simulink model "Expriment_Gaze"  (R2014a)
settings: Solver=FixedStepDiscrete  SolverMode=SingleTasking  StartTime=0.0  StopTime=inf  FixedStep=0.01  RelTol=1e-3
PostLoadFcn:
  | h_RPStest = RPStest;
model workspace (MAT data in the model file):
  gtest = 0
undefined symbols (not defined in the file or in its folder): avert, avert_freq_factor, avert_gaze_dirs_chance, avert_gaze_duration_factor, avert_head_frequency_factor, avert_head_speed, BML, BML1, BML2, bmlsL, bmlsM, bodyBusyFlag, clock, emotion_amount_factor, faceBusyFlag, fileID, GAZE_WIN, gazing, mut_freq_factor, mutual_gaze_duration_factor, P, pose_cat_chance, pose_chanc_factor, pose_chance_factor, pose_frequency_factor, pose_lean, pose_lean_flag, pose_speed, pose_twitch, pr, serial, STATE_BEFORE, STATE_GO, STATE_OVER, STATE_READY, Stateflow
libraries: simulink x24, instrumentlib x6, lib_affectiveChar_behavior x3, realtime_pacer_lib x2, lib_affectiveChar_input x1
(part 7 of 7)

== stateflow chart Expriment_Gaze/CharacterControl/facialExpression_Controller ==
  state subSmile [parallel]
    settings: executionOrder=1
    state stateInitial
      entry: avert=1; gameState=14;
      n=encStr2Arr(' ');bmlsM=[n n n n n];newBmlsM=[n n n n n];
    state stateCheckSmile
    state gazeCamera
      entry:  [P,BMLM]= smileTable(2) ;avert=0;
      newBmlsM=insertQueue(bmlsM,BMLM);
      bmlsM=newBmlsM;
    state wait
    state checkP
      entry:  [P,BMLM]=  smileTable(1) ;
      newBmlsM=insertQueue(bmlsM,BMLM);
      bmlsM=newBmlsM;
    (default) -> stateInitial
    stateInitial -> stateCheckSmile : [gameState==20]
    stateCheckSmile -> stateCheckSmile [order 2]
    gazeCamera -> stateCheckSmile [order 2] : after(1,secs)[isSmiling~=1]
    wait -> stateCheckSmile : after(10,secs)
    stateCheckSmile -> gazeCamera [order 1] : [[isSmiling==1]&[ gameState~= STATE_GO]&[ gameState~= STATE_READY]]
    checkP -> wait
    gazeCamera -> checkP [order 1] : after(1,secs)[isSmiling==1]
  note: SMILE_DUER=10 seceonds
  note: check if still isSmiling is true works as a buffer to remove the smiles that last ony 1 sec (system errors).
  state subFacial [parallel]
    settings: executionOrder=2
    state stateFacialExpression
      entry:
      emotion_amount_factor =set_AU_Amount(inA,inV,personality);
      BMLl=cmdBML_AU_VA(emotion_amount_factor);
      newBmlsL=insertQueueLow(bmlsL,BMLl); bmlsL=newBmlsL;
    state initial
    state wait3
    (default) -> initial
    initial -> stateFacialExpression : [gameState==20]
    wait3 -> stateFacialExpression : after(7,secs)
    stateFacialExpression -> wait3
  data: bmls function_input double size=[1000,5]; myBML function_input double size=[1000,1]; newBmls function_output double size=[1000,5]; bmls function_input double size=[1000,5]; myBML function_input double size=[1000,1]; newBmls function_output double size=[1000,5]; bmlID function_input double; p function_output double size=1; poseBML function_output double size=[1000,1]; bmlID function_input double; p function_output double size=1; poseBML function_output double size=[1000,1]; eAmountFactor function_output double size=[1,11]; arousal function_input double size=1; valence function_input double size=1; inPersonality function_input double size=1; smileN local double size=1; isSmiling input double size=1 =0; avert data_store_memory =0; gazing data_store_memory size=2; GAZE_WIN data_store_memory size=2; BML data_store_memory size=[256,1]; P data_store_memory; fileID local double size=1; gameState output double; STATE_GO data_store_memory; STATE_READY data_store_memory; STATE_BEFORE data_store_memory; newBmlsM local double size=[1000,5]; bmlsM data_store_memory size=[256,1]; BMLM local double size=[1000,1]; n local; personality input double size=1; internalE input double size=1; au local; emotion_amount_factor data_store_memory; aChange input boolean size=1; au_i local double size=1; au_L local double size=1; emoDisp local; bmlsL data_store_memory size=[256,1]; BMLl local double size=[1000,1]; newBmlsL local double size=[1000,5]; emotion_amount_custom input double size=1; inA input double size=1; inV input double size=1; vChange input boolean size=1
  events: secs input RISING_EDGE_EVENT
  function newBmls =insertQueue(bmls,myBML):
    | function newBmls =insertQueue(bmls,myBML)
    |     full=1;
    |     t=encStr2Arr(' ');
    |     newBmls=[t t t t t];
    |     for i = 1:5
    |         if (isequal(bmls(:,i),t))
    |             %add to end of the queue where its empty
    |             bmls(:,i)=myBML;
    |             full=0;
    |             break
    |         end
    |     end
    |     if(full~=0)
    |             %if queue full, shift all elements to left which removes the first one, then add to end
    |             bmls(:,1)= bmls(:,2);
    |             bmls(:,2)= bmls(:,3);
    |             bmls(:,3)= bmls(:,4);
    |             bmls(:,5)=myBML;
    |     end
    |     newBmls=bmls;
  function newBmls =insertQueueLow(bmls,myBML):
    | function newBmls =insertQueueLow(bmls,myBML)
    |     full=1;
    |     t=encStr2Arr(' ');
    |     newBmls=[t t t t t];
    |     for i = 1:5
    |         if (isequal(bmls(:,i),t))
    |             %add to end of the queue where its empty
    |             bmls(:,i)=myBML;
    |             full=0;
    |             break
    |         end
    |     end
    |     if(full~=0)
    |             %if queue full, shift all elements to left which removes the first one, then add to end
    |             bmls(:,1)= bmls(:,2);
    |             bmls(:,2)= bmls(:,3);
    |             bmls(:,3)= bmls(:,4);
    |             bmls(:,5)=myBML;
    |     end
    |     newBmls=bmls;
  function [p,poseBML] = smileTable(bmlID):
    | function [p,poseBML] = smileTable(bmlID)
    | 
    | aVarTruthTableCondition_1 = false;
    | aVarTruthTableCondition_2 = false;
    | 
    | 
    | % smile
    | 
    | aVarTruthTableCondition_1 = logical(bmlID==1);
    | 
    | % headN
    | 
    | aVarTruthTableCondition_2 = logical(bmlID==2);
    | 
    | if (aVarTruthTableCondition_1)
    |     aFcnTruthTableAction_1();
    | elseif (aVarTruthTableCondition_2)
    |     aFcnTruthTableAction_2();
    | else % Default
    |     aFcnTruthTableAction_1();
    | end
    | 
    | function aFcnTruthTableAction_1()
    | 
    | % smile
    | 
    | poseBML=encStr2Arr('<?xml version="1.0"?><act><bml><face amount="1" au="12" side="BOTH" start="0" stroke="2" relax="3" end="4" type="facs"/><face amount="0.3" au="6" side="BOTH" start="0" stroke="2" relax="3" end="4" type="facs"/></bml></act>');p=3;
    | 
    | function aFcnTruthTableAction_2()
    | 
    | % headNeutralBrow
    | 
    | poseBML=encStr2Arr('<?xml version="1.0" ?><act><bml><gaze target="gazeTarget" start="0" end="5" sbm:time-hint="1.5"/></bml></act>');p=3;
    | 
    | function aFcnTruthTableAction_3()
    | 
    | % smileBrow
    | 
    | poseBML=encStr2Arr('<?xml version="1.0"?><act><bml><face amount="0.1" au="1" side="BOTH" start="0" stroke="2" relax="4" end="6" type="facs"/><face amount="0.1" au="2" side="BOTH" start="0" stroke="2" relax="4" end="6" type="facs"/></bml></act>');p=3;
  function [p,poseBML] = facialExpr(bmlID):
    | function [p,poseBML] = facialExpr(bmlID)
    | 
    | aVarTruthTableCondition_1 = false;
    | aVarTruthTableCondition_2 = false;
    | 
    | 
    | % smile
    | 
    | aVarTruthTableCondition_1 = logical(bmlID==1);
    | 
    | % headN
    | 
    | aVarTruthTableCondition_2 = logical(bmlID==2);
    | 
    | if (aVarTruthTableCondition_1)
    |     aFcnTruthTableAction_1();
    | elseif (aVarTruthTableCondition_2)
    |     aFcnTruthTableAction_2();
    | else % Default
    |     aFcnTruthTableAction_1();
    | end
    | 
    | function aFcnTruthTableAction_1()
    | 
    | % smile
    | 
    | poseBML=encStr2Arr('<?xml version="1.0"?><act><bml><face amount="1" au="12" side="BOTH" start="0" stroke="10" relax="70" end="100" type="facs"/><face amount="0.3" au="6" side="BOTH" start="0" stroke="10" relax="70" end="100" type="facs"/></bml></act>');p=3;
    | 
    | function aFcnTruthTableAction_2()
    | 
    | % headNeutralBrow
    | 
    | poseBML=encStr2Arr('<?xml version="1.0" ?><act><bml><gaze target="gazeTarget" start="0" end="5" sbm:time-hint="1.5"/></bml></act>');p=3;
    | 
    | function aFcnTruthTableAction_3()
    | 
    | % smileBrow
    | 
    | poseBML=encStr2Arr('<?xml version="1.0"?><act><bml><face amount="0.1" au="1" side="BOTH" start="0" stroke="2" relax="4" end="6" type="facs"/><face amount="0.1" au="2" side="BOTH" start="0" stroke="2" relax="4" end="6" type="facs"/></bml></act>');p=3;
  function eAmountFactor  =set_AU_Amount(arousal,valence,inPersonality):
    | function eAmountFactor  =set_AU_Amount(arousal,valence,inPersonality)
    | %     15-12-2015, PAD drivern facial expr simul, Grammer data to map AU and VA
    | %     fprintf('VA: %0.0f,%0.0f\r\n',arousal,valence);
    | %     scale
    | %     p = valence * (20/9)  - 10;
    | %     a = arousal * (20/9)  - 10;
    | 
    |     p=valence;a=arousal;
    |     all_AUs=[1,2,4,5,6, 7,12,26,45,10, 25];eAmountFactor=[0,0,0,0,0, 0,0,0,0,0, 0];
    |     for c=1:11
    |         eAmountFactor(1)=0.003*p-0.002*a;  %1,-0.002*a
    |         eAmountFactor(2)=-0.002*p+0.010*a; %2,+0.010*a
    | %         eAmountFactor(12)=-0.016*p+0.034*a; %27 moth open stretch
    |         eAmountFactor(8)=-0.002*p+0.023*a;  %26,-0.002*p+0.049*a
    |         eAmountFactor(5)=-0.008*p+0.009*a;  %6
    |         
    | %         eAmountFactor(13)=0.002*p+0.004*a; %18 lip Puckerer, W 0.3=101
    | %         eAmountFactor(14)=0.007*p+0.025*a; %22 lip fumeler, ShCh 0.5=102       
    | %         eAmountFactor(15)=0.003*p+0.009*a; %14 dimpler FV+PBM 0.5=103
    | %         eAmountFactor(16)=0.003*p+0.009*a; %14 dimpler FV+PBM 0.5=103
    | %         eAmountFactor=-0.010*p+0.017*a;  %17 chin raiser
    | 
    |         eAmountFactor(10)=-0.020*p+0.020*a;  %10 upper lip raiser,-0.053*p+0.026*a
    |         eAmountFactor(4)=-0.003*p+0.032*a; %5 upper lid raiser
    |         eAmountFactor(9)=-0.011*p-0.011*a; %eye closed, 45 instead of 43,-0.021*p-0.037*a
    |         eAmountFactor(3)=-0.036*p+0.022*a; %4 brow lowerer
    | %       eAmountFactor=-0.008*p+0.006*a;    %9 nose wrikler ,10
    | %       eAmountFactor=-0.004*p+0.004*a;    %39?
    | %       eAmountFactor=-0.010*p+0.008*a;    %38?
    | 
    |         eAmountFactor(11)=-0.011*p+0.023*a;%25 lip open,-0.023*p+0.058*a
    | %       eAmountFactor(17)=-0.004*p-0.003*a;    %24 lip pressor, PBM =104       
    | %       eAmountFactor(18)=-0.011*p+0.009*a;    %23 lip tightner PBM0.2 + W0.6=105
    | %       eAmountFactor(19)=-0.011*p+0.009*a;    %23 lip tightner PBM0.2 + W0.6=105
    | 
    | %       eAmountFactor=-0.004*p+0.003*a;    %19?
    | 
    | %       eAmountFactor(20)=0.039*p+0.015*a;  %13 cheek puffer, W 0.3 =106
    |         
    |         eAmountFactor(6)=-0.005*p-0.001*a; %7  Lid Tightener
    |         eAmountFactor(7)=0.057*p+0.009*a;  %12 Lip Corner Puller
    |     %   eAmountFactor=-0.008*p+0.009*a;    %11 Nasolabial Deepener
    |     %   eAmountFactor=-0.046*p-0.002*a;    %15 Lip Corner Depressor
    |     %   eAmountFactor=-0.014*p+0.016*a;    %16 Lower Lip Depressor
    |     %   eAmountFactor(20)=-0.026*p+0.010*a;%20 lip stretch
    |         
    |         eAmountFactor=eAmountFactor/6; %scale
    |         if(inPersonality==2 || inPersonality==4)%introvert
    |             eAmountFactor=eAmountFactor/1.3; % divide by 4/3
    |         end
    |     end

== stateflow chart Expriment_Gaze/GazeFollowSubsystem/reactiveGaze/createGazePawn ==
  state sendBML(In1) [function]
  state sendSBM(In2) [function]
  state stateCreatePawn
    entry:
    sendSBM( encStr2Arr( 'gt = scene.createPawn("gazeTarget")' ) );
    sendBML(encStr2Arr('<?xml version="1.0" ?><act><bml><gaze sbm:joint-range="EYES BACK" target="gazeTarget"/></bml></act>'));
  (default) -> stateCreatePawn
  data: In1 function_input double size=[1000 1]; In2 function_input double size=[1000 1]

== matlab function Expriment_Gaze/randomArray/makleArray ==
  data: r1 input; y output double size=[1,25]; r2 input; r3 input; r4 input; r5 input; r6 input; r7 input; r8 input; r9 input; r10 input; r11 input; r12 input; r13 input; r14 input; r15 input; r16 input; r17 input; r18 input; r19 input; r20 input; r21 input; r22 input; r23 input; r24 input; r25 input
function y = fcn(r1,r2,r3,r4,r5,r6,r7,r8,r9,r10,r11,r12,r13,r14,r15,r16, r17, r18, r19,r20,r21,r22,r23,r24,r25)
%#codegen
y=[0,0,0,0,0,0,0,0,0,0,0,0,0,0,0,0,0,0,0,0,0,0,0,0,0];
y(:,1) = floor(r1);
y(:,2) = floor(r2);
y(:,3) = floor(r3);
y(:,4) = floor(r4);
y(:,5) = floor(r5);
y(:,6) = floor(r6);
y(:,7) = floor(r7);
y(:,8) = floor(r8);
y(:,9) = floor(r9);
y(:,10) = floor(r10);
y(:,11) = floor(r11);
y(:,12) = floor(r12);
y(:,13) = floor(r13);
y(:,14) = floor(r14);
y(:,15) = floor(r15);
y(:,16) = floor(r16);
y(:,17) = floor(r17);
y(:,18) = floor(r18);
y(:,19) = floor(r19);
y(:,20) = floor(r20);
y(:,21) = floor(r21);
y(:,22) = floor(r22);
y(:,23) = floor(r23);
y(:,24) = floor(r24);
y(:,25) = floor(r25);

== matlab function Expriment_Gaze/GazeFollowSubsystem/gazeFollow ==
  data: state input; stateOver output
function stateOver = fcn(state)
%#codegen

%Maryam 30/06/2015
%Here set in which states of the interaction agent experienced 
% more arousal(arousalFlag=1) and less arousal (arousalFlag=-1)

%Note that you should define the states in your scenraio beforehand

%we assume agent gets more aroused when in ready/go state and 
%less aroused when in WAITE/HAND

if(state==3)%only gaze follows user in ganme-over states 
                      %since in other states we assume user is not moving
    stateOver=1;
else
    stateOver=0;

end

== matlab function Expriment_Gaze/handUpTable ==
  data: R input; L input; y output
function y = fcn(R, L)

aVarTruthTableCondition_1 = false;
aVarTruthTableCondition_2 = false;
aVarTruthTableCondition_3 = false;
aVarTruthTableCondition_4 = false;


% no hand up

aVarTruthTableCondition_1 = logical(R==0 && L==0);

% right hand up

aVarTruthTableCondition_2 = logical(R==1 && L==0);

% left hand up

aVarTruthTableCondition_3 = logical(R==0 && L==1);

% both hands up

aVarTruthTableCondition_4 = logical(R==1 && L==1);

if (aVarTruthTableCondition_1)
    aFcnTruthTableAction_1();
elseif (aVarTruthTableCondition_2)
    aFcnTruthTableAction_2();
elseif (aVarTruthTableCondition_3)
    aFcnTruthTableAction_3();
elseif (aVarTruthTableCondition_4)
    aFcnTruthTableAction_4();
else % Default
    aFcnTruthTableAction_1();
end

function aFcnTruthTableAction_1()

% no hand up

y = 0;

function aFcnTruthTableAction_2()

% right hand up

y = 1;

function aFcnTruthTableAction_3()

% left hand up

y = 2;

function aFcnTruthTableAction_4()

% both hands up

y = 3;

== matlab function Expriment_Gaze/facialExpr/facialExprGen/setAU ==
  data: E input double size=1; AU output double size=[1,6]; L output double size=1
function [AU,L]=setAU(E)	
% 1	Inner Brow Raiser,% 2	Outer Brow Raiser, % 4	Brow Lowerer
% 5	Upper Lid Raiser,% 6	Cheek Raiser,% 7	Lid Tightener
% 8	Lips Toward Each Other,% 9	Nose Wrinkler,% 10	Upper Lip Raiser	
% 11	Nasolabial Deepener	% 12	Lip Corner Puller % 13	Sharp Lip Puller % 14	Dimpler	
% 15	Lip Corner Depressor % 16	Lower Lip Depressor % 17	Chin Raiser	mentalis
% 18	Lip Pucker	% 19	Tongue Show	% 20	Lip Stretcher % 21	Neck Tightener	platysma
% 22	Lip Funneler% 23	Lip Tightener% 24	Lip Pressor % 25	Lips Part	depressor
% 26	Jaw Drop,% 27	Mouth Stretch
% 43	Eyes Closed, % 44	Eyebrow Gatherer,% 45	Blink,% 46	Wink
%smartbody no 43,15,17,10 looks wierd,no 142
   AU=[6,12,142,0,0,0];L=3;
   % AU5(eyeOpen) for A+
   % AU1,4 for V-
   %AU12 for V+
    switch(E)
        case 1 %V- A-,bored (43)[1]
            AU=[1,2,45,0,0,0];L=3;%[1,1,0.35]
        
        case 2 %V- A-;sad %(1,2,4,10,15,17,43)[];can be [1,2,4,45,6,0]
            AU=[1,4,0,0,0,0];L=2;%[1,1,0,0,0,0]
        
        case 3 %V- A+,frust(2,1,14)[1],(-1,-2,4,7,14)[2], maybe(1,7)[0.7,0.7,0.5]
            AU=[1,2,4,5,6,0];L=5;%[1,1,1,0.5,0.5,0]
        
        case 4 %V- A+,fear(1,2,4,5,25=mouth)
            AU=[1,2,4,5,6,7];L=6; %[1,1,1,0.2,0.2]
        
        case 5%V+ A-,calm,sleepy
            AU=[12,14,0,0,0,0];L=2;%[0.7,0.3,0,0,0,0]
        
        case 7%V+ A+,happy
            AU=[6,12,0,0,0,0];L=2;%[1,0.5,0,0,0,0]
        
        case 8%V+ A+,excited
            AU=[12,26,5,1,2,0];L=5;%[1,1,1,1,1,0]
        
        case 9%V- A+, angry
            AU=[2,4,5,7,45,0];L=5;%[0.5,1,0.2,0.2,0.2]
        
        otherwise
            %confusion (1,2,4,7)[1] %[1,1,1,0.2]
            %worried (1,2,4,5) [1,1,1,0.5]
            %angry(4,5,7,10,27)[], can be(2,4,5,7,45)[0.5,1,0.2,0.2,0.2]

            AU=[4,7,12,0,0,0];L=3;
            disp('error, emotion not listed:');disp(E);
    end  
%[1]Craig S.D. et al(2004)emotions during learning:the first steps tw affect sensitive
%[2]grafsgard J F () automatically recog facial indicator of frust

== matlab function Expriment_Gaze/facialExpr/facialExprGen/forloop/displayBMLs ==
  data: e input; l input; i input double size=1 [1..]; bml input
function fcn(e,l,i,bml)
%#codegen
fprintf('%s','e:');fprintf('%f',e);
fprintf('%s','  ,L:');fprintf('%f',l);
fprintf('%s','  ,i:');fprintf('%f',i);
disp(decArr2Str(bml));

== matlab function Expriment_Gaze/readSHORE/smile/ifSmile ==
  data: u input; y output
function y = fcn(u)
%#codegen
if u>0.5
    smile=1;
else
    smile=0;
end
y = smile;

== matlab function Expriment_Gaze/facialExpr/facialExprGen/setAmount ==
  data: E input double size=1; eAmountFactor output double size=[1,6]; Pt input double size=1
function eAmountFactor =setAmount(E,Pt)
    AU=[6,12,142,0,0,0];eAmountFactor=[1,1,1,0,0,0];pFactor=1;
    
    if(Pt==1)
        %HEHN
        if(E==1)  %bored
            eAmountFactor=[1,1,0,0.35,0,0];
        elseif(E==2) %sad
            eAmountFactor=[1,1,0,0,0,0];
        elseif(E==3) %frust
            eAmountFactor=[1,1,1,0.5,0.5,0];
        elseif(E==4) %fear
            eAmountFactor=[1,1,1,0.2,0.2,0];
        elseif(E==5)%sleepy
            eAmountFactor=[0.7,0.3,0.3,0,0,0];
        elseif(E==7)%happy
            eAmountFactor=[1,0.5,0,0,0,0];
        elseif(E==8)%excited
            eAmountFactor=[1,1,1,1,1,0];    
        else          
            eAmountFactor=[1,1,1,0,0,0];
            disp('error, emotion not listed:');disp(E);
        end
    
        %LEHN  
    elseif(Pt==2)
       if(E==1)  %bored
            eAmountFactor=[1,1,0,0.35,0,0];
        elseif(E==2) %sad
            eAmountFactor=[1,1,0,0,0,0];
        elseif(E==3) %frust
            eAmountFactor=[1,1,1,0.5,0.5,0];
        elseif(E==4) %fear
            eAmountFactor=[1,1,1,0.2,0.2,0];
        elseif(E==5)%sleepy
            eAmountFactor=[0.7,0.3,0.3,0,0,0];
        elseif(E==7)%happy
            eAmountFactor=[1,0.5,0,0,0,0];
        elseif(E==8)%excited
            eAmountFactor=[1,1,1,1,1,0];    
        else          
            eAmountFactor=[1,1,1,0,0,0];
            disp('error, emotion not listed:');disp(E);
        end

        %HELN
   elseif(Pt==3)
        if(E==1)  %bored
            eAmountFactor=[1,1,0,0.35,0,0];
        elseif(E==2) %sad
            eAmountFactor=[1,1,0,0,0,0];
        elseif(E==3) %frust
            eAmountFactor=[1,1,1,0.5,0.5,0];
        elseif(E==4) %fear
            eAmountFactor=[1,1,1,0.2,0.2,0];
        elseif(E==5)%sleepy
            eAmountFactor=[0.7,0.3,0.3,0,0,0];
        elseif(E==7)%happy
            eAmountFactor=[1,0.5,0,0,0,0];
        elseif(E==8)%excited
            eAmountFactor=[1,1,1,1,1,0];    
        else          
            eAmountFactor=[1,1,1,0,0,0];
            disp('error, emotion not listed:');disp(E);
        end
        eAmountFactor=eAmountFactor*pFactor;
        %LELN
    elseif(Pt==4)
        if(E==1)  %bored
            eAmountFactor=[1,1,0,0.35,0,0];
        elseif(E==2) %sad
            eAmountFactor=[1,1,0,0,0,0];
        elseif(E==3) %frust
            eAmountFactor=[1,1,1,0.5,0.5,0];
        elseif(E==4) %fear
            eAmountFactor=[1,1,1,0.2,0.2,0];
        elseif(E==5)%sleepy
            eAmountFactor=[0.7,0.3,0.3,0,0,0];
        elseif(E==7)%happy
            eAmountFactor=[1,0.5,0,0,0,0];
        elseif(E==8)%excited
            eAmountFactor=[1,1,1,1,1,0];    
        else          
            eAmountFactor=[1,1,1,0,0,0];
            disp('error, emotion not listed:');disp(E);
        end
        eAmountFactor=eAmountFactor*pFactor;
    end
%Following is if we want a same factor for each personaliy all through AUs
% function eAmountFactor =set_eAmountFactor(E,P)
%     AU=[6,12,142,0,0,0];eAMOUNT=[0,0,0,0,0,0];
%     switch E
%         case 1  %bored
%             eAMOUNT=[1,1,1,0,0,0];
%         case 2 %sad
%             eAMOUNT=[0.7,0.4,0.9,0,0,0];
%         case 3 %angry
%             eAMOUNT=[1,0.8,1,0,0,0];
%         case 4 %fear
%             eAMOUNT=[1,1,1,0,0,0];%5,6,7,26
%         case 5%contempt
%             eAMOUNT=[1,1,1,0,0,0];
%         case 7%happy
%             eAMOUNT=[0.2,1,0,0,0,0];
%         otherwise           
%             eAMOUNT=[0,0,0,0,0,0];
%             disp('error,amount for emotion not listed:');disp('eAMOUNT');
%     end 
%     switch P
%         case 1 %HEHN
%             pFactor=1;
%         case 2 %LEHN
%             pFactor=1;
%         case 3 %HELN
%             pFactor=0.5;
%         case 4 %LELN
%             pFactor=0.5;
%     end
%     eAmountFactor=pFactor*eAMOUNT;

== matlab function Expriment_Gaze/facialExpr/facialExprGen/emotionBMLsLoop/displayBMLs ==
  data: e input; i input double size=1 [1..]; bml input
function fcn(e,i,bml)
%#codegen
fprintf('%f',e);
fprintf('%d',i);
disp(decArr2Str(bml));

== matlab function Expriment_Gaze/facialExpr/facialExprGen/emotionBMLsLoop/loopInBmls ==
  data: i input double size=1 [1..]; arrAU input; eAmount input; arrBML output
function arrBML = fcn(i,arrAU,eAmount)
    %#codegen
    coder.extrinsic('sprintf');
    coder.extrinsic('strcat');
    
    %Maryam, 14-10-2015
    %'strcat' dimension 2  maximum size is 453,it was not possible to concat and send all bmls 
    %for one emotion together(used simulink for loop )    
    
    AU=arrAU(i);eA=eAmount(i);   
    c1 = countDigits(AU);c2 = countDigits(eA);

    str1 = sprintf('<?xml version=\"1.0\" ?><act><bml>');
    
    if(max(ceil(log10(abs(AU))),1)==1) %if AU is one-digit
        temp = sprintf('<face type=\"FACS\" side=\"BOTH\" au=\"%1d\"  start=\"0\" end=\"3\" amount=\"%0.1f\"/>',AU,eA); 
        temp2=strcat(str1,temp);
        str1=temp2;
    else      
        temp = sprintf('<face type=\"FACS\" side=\"BOTH\" au=\"%2d\"  start=\"0\" end=\"3\" amount=\"%0.1f\"/>',AU,eA);
        temp2=strcat(str1,temp);
        str1=temp2;
    end

    str2 = sprintf('</bml></act>');
    %n=length(arrAU);
    %mystr=blanks(arrAU(n));
    mystr=blanks(140+c1+c2);
    mystr = strcat (str1,str2);    
    arrBML = encStr2Arr(mystr);

== matlab function Expriment_Gaze/facialExpr/facialExprGen/forloop/makeBmlsFor ==
  data: i input double size=1 [1..]; arrAU input; eAmount input; arrBML1 output; arrBML2 output; arrBML3 output; arrBML4 output; arrBML5 output; arrBML6 output
function [arrBML1,arrBML2,arrBML3,arrBML4,arrBML5,arrBML6] = fcn(i,arrAU,eAmount)
    %#codegen
    coder.extrinsic('sprintf');
    coder.extrinsic('strcat');
    arrBML1=encStr2Arr('');arrBML2=encStr2Arr('');arrBML3=encStr2Arr('');
    arrBML4=encStr2Arr('');arrBML5=encStr2Arr('');arrBML6=encStr2Arr('');
    %Maryam, 14-10-2015
    %'strcat' dimension 2  maximum size is 453,it was not possible to concat and send all bmls 
    %for one emotion together(used simulink for loop )    
    
    AU=arrAU(i);eA=eAmount(i);   
    c1 = countDigits(AU);c2 = countDigits(eA);

    str1 = sprintf('<?xml version=\"1.0\" ?><act><bml>');
    
    if(max(ceil(log10(abs(AU))),1)==1) %if AU is one-digit
        temp = sprintf('<face type=\"FACS\" side=\"BOTH\" au=\"%1d\"  start=\"0\" ready=\"1\" stroke=\"2\"  relax=\"3\" end=\"4\" amount=\"%0.1f\"/>',AU,eA); 
        temp2=strcat(str1,temp);
        str1=temp2;
    else      
        temp = sprintf('<face type=\"FACS\" side=\"BOTH\" au=\"%2d\" start=\"0\" ready=\"1\" stroke=\"2\"  relax=\"3\" end=\"4\" amount=\"%0.1f\"/>',AU,eA);
        temp2=strcat(str1,temp);
        str1=temp2;
    end

    str2 = sprintf('</bml></act>');
    %n=length(arrAU);
    %mystr=blanks(arrAU(n));
    mystr=blanks(140+c1+c2);
    mystr = strcat (str1,str2);  
    if(i==1)
        arrBML1 = encStr2Arr(mystr);
    elseif(i==2)
        arrBML2 = encStr2Arr(mystr);
     elseif(i==3)
            arrBML3 = encStr2Arr(mystr);
     elseif(i==4)
            arrBML4 = encStr2Arr(mystr);
     elseif(i==5)
            arrBML5 = encStr2Arr(mystr);
     elseif(i==6)
            arrBML6 = encStr2Arr(mystr);
    end

== matlab function Expriment_Gaze/facialExpr/facialExprGen/forloop1/displayBMLs ==
  data: e input; l input; i input double size=1 [1..]; bml input
function fcn(e,l,i,bml)
%#codegen
fprintf('%s','e:');fprintf('%f',e);
fprintf('%s','  ,L:');fprintf('%f',l);
fprintf('%s','  ,i:');fprintf('%f',i);
disp(decArr2Str(bml));

== stateflow chart Expriment_Gaze/GazeFollowSubsystem/resetGazeTarget/createGazePawn ==
  state sendSBM(In2) [function]
  state stateCreatePawn
    entry:
    sendSBM(encStr2Arr('scene.getPawn(\"gazeTarget\").setPosition(SrVec(0,1.6,10))'));
  (default) -> stateCreatePawn
  data: In2 function_input double size=[1000 1]

== matlab function Expriment_Gaze/chack_E_Change1/checkNeutral ==
  data: notNeutral output double size=1; e input
function notNeutral = fcn(e)
%#codegen

if(e~=6)
    notNeutral=1;
else
    notNeutral=0;
end

== matlab function Expriment_Gaze/setPersonality ==
  data: extrovert input; personality output; neurotic input
function personality = fcn(extrovert,neurotic)
%#codegen
% 1 HEHN 2 LEHN 3 HELN 4 LELN
if(extrovert==1)
    if(neurotic==1)
        personality = 1;% 1 HEHN
    else 
        personality = 3;%HELN
    end
else
    if(neurotic==1)
        personality = 2;%LEHN
    else
        personality = 4;%LELN
    end
end

== matlab function Expriment_Gaze/EmotionSubsystem/calculateValenceArousal/HEHN_VA_Emo ==
  data: V input; e output double size=1; A input double
function e = fcn(V, A)

aVarTruthTableCondition_1 = false;
aVarTruthTableCondition_2 = false;
aVarTruthTableCondition_3 = false;
aVarTruthTableCondition_4 = false;
aVarTruthTableCondition_5 = false;
aVarTruthTableCondition_6 = false;
aVarTruthTableCondition_7 = false;
aVarTruthTableCondition_8 = false;


% 7-happy  2,1

aVarTruthTableCondition_1 = logical(V>10 && A<40 && A>10);

% 8-ex  1,2 AND 2,2

aVarTruthTableCondition_2 = logical(V>0 && A>40);

% 4-fear  -1,2 AND -2,2

aVarTruthTableCondition_3 = logical(V<0 && A>40);

% 3-frust  -2,1

aVarTruthTableCondition_4 = logical(V<-10 && A<40 && A>10);

% 6-pleased  2,-1

aVarTruthTableCondition_5 = logical(V>10 && A<-10 && A>-40);

% 5-calm  1,-2 AND 2,-2

aVarTruthTableCondition_6 = logical(V>0 && A<-40);

% 1-bored  -1,-2 AND -2,-2

aVarTruthTableCondition_7 = logical(V<0 && A<-40);

% 2-sad  -2,-1

aVarTruthTableCondition_8 = logical(V<-10 && A<-10 && A>-40);

if (aVarTruthTableCondition_1)
    aFcnTruthTableAction_1();
elseif (aVarTruthTableCondition_2)
    aFcnTruthTableAction_2();
elseif (aVarTruthTableCondition_3)
    aFcnTruthTableAction_3();
elseif (aVarTruthTableCondition_4)
    aFcnTruthTableAction_4();
elseif (aVarTruthTableCondition_5)
    aFcnTruthTableAction_5();
elseif (aVarTruthTableCondition_6)
    aFcnTruthTableAction_6();
elseif (aVarTruthTableCondition_7)
    aFcnTruthTableAction_7();
elseif (aVarTruthTableCondition_8)
    aFcnTruthTableAction_8();
else % Default
    aFcnTruthTableAction_5();
end

function aFcnTruthTableAction_1()

% happy

e=7;

function aFcnTruthTableAction_2()

% excited

e=8;

function aFcnTruthTableAction_3()

% fear

e=4;

function aFcnTruthTableAction_4()

% frustration

e=3;

function aFcnTruthTableAction_5()

% pleased

e=6;

function aFcnTruthTableAction_6()

% contempt

e=5;

function aFcnTruthTableAction_7()

% bored

e=1;

function aFcnTruthTableAction_8()

% sad

e=2;

== matlab function Expriment_Gaze/gazeInputArray/makeGazeArray ==
  data: r1 input; y output double size=[1,6]; r2 input; r3 input; r4 input; r5 input; r6 input
function y = fcn(r1,r2,r3,r4,r5,r6)
%#codegen
y=[0,0,0,0,0,0];
y(:,1) = floor(r1);
y(:,2) = floor(r2);
y(:,3) = floor(r3);
y(:,4) = floor(r4);
y(:,5) = floor(r5);
y(:,6) = floor(r6);

== stateflow chart Expriment_Gaze/CharacterControl/personality_Behavior_Factors ==
  state setP
    entry:
    [mutual_gaze_duration_factor, avert_gaze_duration_factor,avert_head_frequency_factor,avert_head_speed,avert_gaze_dirs_chance,avert_freq_factor,mut_freq_factor,blink_flag, blinkperiod_min,blinkperiod_max]=sharedFunc.setGazeFactors(inV,inA,personality,personalityFlag,vaFlag,gazeArray);
    %[pose_twitch,pose_frequency_factor,pose_chanc_factor,pose_cat_chance,pose_lean,pose_speed,pose_lean_flag]=sharedFunc.setPoseFactors(inV,inA,personality,personalityFlag,vaFlag,poseArray,personalityChange);
  state init
    entry: mutual_gaze_duration_factor=1;avert_gaze_duration_factor=1;,avert_freq_factor=1;mut_freq_factor=1;
    avert_head_frequency_factor=20;avert_head_speed=1;avert_gaze_dirs_chance=1;blink_flag=0; blinkperiod_min=5;blinkperiod_max=9;
    pose_lean_flag=0; pose_frequency_factor=20;pose_chanc_factor=1;pose_cat_chance=70;pose_lean=10;pose_speed=1;
  state wait
  state sharedFunc [group]
  (default) -> init
  wait -> setP : [personalityChange==1]
  setP -> wait
  init -> wait
  data: inA input double size=1; inV input double size=1; vaFlag input boolean size=1; personalityFlag input boolean size=1; gazeArray input double size=[1, 6]; personality input double size=1; personalityChange input boolean size=1; mutual_gaze_duration_factor data_store_memory; avert_head_frequency_factor data_store_memory; avert_gaze_duration_factor data_store_memory; avert_head_speed data_store_memory; avert_gaze_dirs_chance data_store_memory; poseArray input double size=[1, 6]; pose_chanc_factor data_store_memory; pose_frequency_factor data_store_memory; pose_lean data_store_memory; pose_change_flag data_store_memory; pose_lean_flag data_store_memory; pose_speed data_store_memory; pose_cat_chance data_store_memory; internalE input double size=1; emotion_amount_custom input double size=1; emotion_amount_factor data_store_memory size=1; mut_freq_factor data_store_memory; avert_freq_factor data_store_memory; pose_twitch data_store_memory; blinkperiod_min data_store_memory; blink_flag data_store_memory; blinkperiod_max data_store_memory

== stateflow chart Expriment_Gaze/CharacterControl/custom_Behavior_Factors ==
  state setP
    entry:
    [mutual_gaze_duration_factor, avert_gaze_duration_factor,avert_head_frequency_factor,avert_head_speed,avert_gaze_dirs_chance,avert_freq_factor,mut_freq_factor]=sharedFunc.setGazeFactors(inV,inA,personality,personalityFlag,vaFlag,gazeArray);
  state init
    entry: mutual_gaze_duration_factor=1;avert_gaze_duration_factor=1;
    avert_head_frequency_factor=1;avert_head_speed=1;avert_gaze_dirs_chance=1;,avert_freq_factor=1;mut_freq_factor=1;
    pose_frequency_factor=5;pose_chanc_factor=1;pose_cat_chance=10;pose_lean=10;pose_speed=1;pose_lean_flag=0;
  state wait
  state sharedFunc [group]
  state setP1
    entry:
    [pose_twitch,pose_frequency_factor,pose_chanc_factor,pose_cat_chance,pose_lean,pose_speed,pose_lean_flag]=sharedFunc.setPoseFactors(inV,inA,personality,personalityFlag,vaFlag,poseArray,personalityChange);
  (default) -> init
  init -> wait
  setP -> wait
  wait -> setP [order 1] : [gazeArray(:,1)==1]
  setP1 -> wait
  wait -> setP1 [order 2] : [poseArray(:,1)==1]
  data: inA input double size=1; inV input double size=1; vaFlag input boolean size=1; personalityFlag input boolean size=1; gazeArray input double size=[1, 6]; personality input double size=1; personalityChange input boolean size=1; mutual_gaze_duration_factor data_store_memory; avert_head_frequency_factor data_store_memory; avert_gaze_duration_factor data_store_memory; avert_head_speed data_store_memory; avert_gaze_dirs_chance data_store_memory; poseArray input double size=[1, 6]; pose_lean data_store_memory; pose_speed data_store_memory; pose_chanc_factor data_store_memory; pose_frequency_factor data_store_memory; pose_cat_chance data_store_memory; pose_lean_flag data_store_memory; emotion_amount_custom input double size=1; emotion_amount_factor data_store_memory size=1; mut_freq_factor data_store_memory; avert_freq_factor data_store_memory; pose_twitch data_store_memory

== matlab function Expriment_Gaze/EmotionSubsystem/calculateValenceArousal/HELN plot ==
  data: v input; a input
function fcn(v,a)
%coder.extrinsic to bypass code generation
coder.extrinsic('fscanf')
coder.extrinsic('get_param');
% coder.extrinsic('importdata');

currentTime=get_param('Expriment_FacialExpr','SimulationTime');%use name of simulink proj

A = [v;a;currentTime];

fileID = fopen('HELN_VA_table.txt','a');
fprintf(fileID,'%0.1f,%0.1f,%0.1f\r\n',A);
fclose(fileID);

%use the following to draw the plot
%tmp_data = importdata('HEHN_VA_table.txt',','); 
%no need: x=tmp_data(:,1);y=tmp_data(:,2);z=tmp_data(:,3)
%matrix=tmp_data
%tri = delaunay(matrix(:,1),matrix(:,2));
%trisurf(tri,matrix(:,1),matrix(:,2),matrix(:,3))
%shading interp

%-----------------------------------------
% fileID = fopen('HEHN_VA_table.txt','r');
% formatSpec = '%1f\r %1f\r %1f\r\n';
% sizeA = [3 Inf];
% A = fscanf(fileID,formatSpec,sizeA)
% % A = A'
% fclose(fileID);

% x = zeros(100,2);y = zeros(100,2);
% filename = 'HEHN_VA_table.txt';
% delimiterIn = ' ';
% headerlinesIn = 1;
% A = importdata(filename,delimiterIn,headerlinesIn);

% fileID=fopen('HEHN_VA_table4.txt');
% s=textscan(fileID,'%d %d %d','headerlines',23);
% fclose(fileID);
% x=s{1}

== matlab function Expriment_Gaze/EmotionSubsystem/calculateValenceArousal/HEHN_V ==
  data: v2 output double size=1; v1 input double size=1
function v2 = fcn(v1)

aVarTruthTableCondition_1 = false;
aVarTruthTableCondition_2 = false;



aVarTruthTableCondition_1 = logical(v1>10);


aVarTruthTableCondition_2 = logical(v1<-10);

if (aVarTruthTableCondition_1)
    aFcnTruthTableAction_1();
elseif (aVarTruthTableCondition_2)
    aFcnTruthTableAction_2();
else % Default
    aFcnTruthTableAction_3();
end

function aFcnTruthTableAction_1()


v2=v1;

function aFcnTruthTableAction_2()


v2=v1;

function aFcnTruthTableAction_3()


v2=0;

== matlab function Expriment_Gaze/EmotionSubsystem/calculateValenceArousal/LEHN_V ==
  data: v2 output double size=1; v1 input double size=1
function v2 = fcn(v1)

aVarTruthTableCondition_1 = false;
aVarTruthTableCondition_2 = false;



aVarTruthTableCondition_1 = logical(v1>25);


aVarTruthTableCondition_2 = logical(v1<-25);

if (aVarTruthTableCondition_1)
    aFcnTruthTableAction_1();
elseif (aVarTruthTableCondition_2)
    aFcnTruthTableAction_2();
else % Default
    aFcnTruthTableAction_3();
end

function aFcnTruthTableAction_1()


v2=v1;

function aFcnTruthTableAction_2()


v2=v1;

function aFcnTruthTableAction_3()


v2=0;

== matlab function Expriment_Gaze/EmotionSubsystem/calculateValenceArousal/LELN_A ==
  data: a2 output double size=1; a1 input double size=1
function a2 = fcn(a1)

aVarTruthTableCondition_1 = false;
aVarTruthTableCondition_2 = false;



aVarTruthTableCondition_1 = logical(a1>25);


aVarTruthTableCondition_2 = logical(a1<-25);

if (aVarTruthTableCondition_1)
    aFcnTruthTableAction_1();
elseif (aVarTruthTableCondition_2)
    aFcnTruthTableAction_2();
else % Default
    aFcnTruthTableAction_3();
end

function aFcnTruthTableAction_1()


a2=a1;

function aFcnTruthTableAction_2()


a2=a1;

function aFcnTruthTableAction_3()


a2=0;

== matlab function Expriment_Gaze/EmotionSubsystem/calculateValenceArousal/LELN_VA_Emo ==
  data: V input; e output double size=1; A input double
function e = fcn(V, A)

aVarTruthTableCondition_1 = false;
aVarTruthTableCondition_2 = false;
aVarTruthTableCondition_3 = false;
aVarTruthTableCondition_4 = false;
aVarTruthTableCondition_5 = false;
aVarTruthTableCondition_6 = false;
aVarTruthTableCondition_7 = false;
aVarTruthTableCondition_8 = false;


% 7-happy  2,1

aVarTruthTableCondition_1 = logical(V>20 && A<40 && A>20);

% 8-ex  1,2 AND 2,2

aVarTruthTableCondition_2 = logical(V>0 && A>40);

% 4-fear  -1,2 AND -2,2

aVarTruthTableCondition_3 = logical(V<0 && A>40);

% 3-frust  -2,1

aVarTruthTableCondition_4 = logical(V<-20 && A<40 && A>20);

% 6-idle  2,-1

aVarTruthTableCondition_5 = logical(V>20 && A<-20 && A>-40);

% 5-calm  1,-2 AND 2,-2

aVarTruthTableCondition_6 = logical(V>0 && A<-40);

% 1-bored  -1,-2 AND -2,-2

aVarTruthTableCondition_7 = logical(V<0 && A<-40);

% 2-sad  -2,-1

aVarTruthTableCondition_8 = logical(V<-20 && A<-20 && A>-40);

if (aVarTruthTableCondition_1)
    aFcnTruthTableAction_1();
elseif (aVarTruthTableCondition_2)
    aFcnTruthTableAction_2();
elseif (aVarTruthTableCondition_3)
    aFcnTruthTableAction_3();
elseif (aVarTruthTableCondition_4)
    aFcnTruthTableAction_4();
elseif (aVarTruthTableCondition_5)
    aFcnTruthTableAction_5();
elseif (aVarTruthTableCondition_6)
    aFcnTruthTableAction_6();
elseif (aVarTruthTableCondition_7)
    aFcnTruthTableAction_7();
elseif (aVarTruthTableCondition_8)
    aFcnTruthTableAction_8();
else % Default
    aFcnTruthTableAction_5();
end

function aFcnTruthTableAction_1()

% happy

e=7;

function aFcnTruthTableAction_2()

% excited

e=8;

function aFcnTruthTableAction_3()

% fear

e=4;

function aFcnTruthTableAction_4()

% frustration

e=3;

function aFcnTruthTableAction_5()

% idle

e=6;

function aFcnTruthTableAction_6()

% contempt

e=5;

function aFcnTruthTableAction_7()

% bored

e=1;

function aFcnTruthTableAction_8()

% sad

e=2;

== matlab function Expriment_Gaze/EmotionSubsystem/satFunction ==
  data: randv input; smile input; wave input; win input; invade input; v_trigW output; vaFlag input; v_trig output
function [v_trigW,v_trig]= fcn(randv,smile,wave,win,invade,vaFlag)
%#codegen
% 30/06/2015
    %Here set Agent's satisfaction flag based on your scenario
    %In RPS scenario agent gets satisfined when she wins. states of interaction= {STATE_READY=7;
    %STATE_GO=1;STATE_HAND=2;STATE_OVER=3; STATE_BEFORE=4;STATE_RESULT=5;STATE_WAIT=6;}
   
    if(vaFlag==1)
        v_trigW=0;%weight by which valence value is changed (sum of weight of all triggers)
        %randv 30% chance of random increase or decrease in valence
        randTrigger=floor(randv);
        if(0<randTrigger)&&(randTrigger<30)
            v_trigW = v_trigW + 0.6;
        end
        if(30<randTrigger)&&(randTrigger<60)
            v_trigW = v_trigW - 0.6;
        end

        if(win==2) %agent wins so she is satisfied
            v_trigW = v_trigW + 0.5;
        elseif(win==1) %user wins so agent is NOT satisfied
            v_trigW = v_trigW - 0.5;
        end

        if(smile==1)
            v_trigW=v_trigW+0.25;
        end

        if(wave==1)
            v_trigW=v_trigW+0.25;
        end

        if(invade==1)
            v_trigW=v_trigW-0.25;
        end
    else
         v_trigW=0;
    end
    if(v_trigW>0)
        v_trig=1;
    elseif(v_trigW<0)
        v_trig=-1;
        v_trigW=abs(v_trigW);
    else
        v_trig=0;
    end
